simulink model "Simul_BASE_XLS"  (Simulink 9.0)
settings: Solver=FixedStepAuto  StartTime=0.0  StopTime=140  FixedStep=0.1  RelTol=1e-3  EnableMultiTasking=on
values from neighbouring files (symbols this model uses):
  attitude_0 = [0,0,0]    [ga_detumbling.m]    (also in ga_detumbling_fit.m = [0.0524,-0.0349,0.0175]; ga_pid.m; ga_pid_fit.m; ga_pid_test.m)
  attitude_rate_0 = [0,6.7e-05,0.0041]    [ga_detumbling.m]    (also in ga_detumbling_fit.m = [0.0873,-0.0873,-0.0873]; ga_pid.m; ga_pid_fit.m; ga_pid_test.m)
  dp = x(2)    [ga_detumbling.m]    (also in ga_detumbling_fit.m = d(2); ga_pid.m = x(4); ga_pid_fit.m = d(4); ga_pid_test.m = x(4))
  dr = x(1)    [ga_detumbling.m]    (also in ga_detumbling_fit.m = d(1); ga_pid.m = x(2); ga_pid_fit.m = d(2); ga_pid_test.m = x(2))
  dy = x(3)    [ga_detumbling.m]    (also in ga_detumbling_fit.m = d(3); ga_pid.m = x(6); ga_pid_fit.m = d(6); ga_pid_test.m = x(6))
  override = 2    [ga_pid_fit.m]    (also in ga_pid_test.m; init_var.m)
  pp = x(3)    [ga_pid.m]    (also in ga_pid_fit.m = d(3); ga_pid_test.m; init_var.m = 0.6885)
  pr = x(1)    [ga_pid.m]    (also in ga_pid_fit.m = d(1); ga_pid_test.m; init_var.m = 0.8646)
  py = x(5)    [ga_pid.m]    (also in ga_pid_fit.m = d(5); ga_pid_test.m; init_var.m = 0.371)
  slew = [60 0 0]    [ga_detumbling.m]    (also in ga_pid.m; ga_pid_fit.m; ga_pid_test.m)
libraries: simulink_extras x14, aerolibanim x1, sharedutil x1
CloseFcn:
  | rtwprivate ssgencode ModelCloseRequest Simul_BASE_3MW
settings Model: Creator=Kendrick  LastModifiedBy=bjt
settings SolverCC: MaxConsecutiveMinStep=5  ZeroCrossAlgorithm=Adaptive
settings DataIOCC: LimitDataPoints=on
settings OptimizationCC: ExpressionDepthLimit=2147483647
settings DebuggingCC: AlgebraicLoopMsg=none  SolverPrmCheckMsg=warning  FcnCallInpInsideContextMsg=warning  StateNameClashWarn=warning
settings HardwareCC: ProdBitPerInt=16  ProdBitPerPointer=16  ProdBitPerSizeT=16  ProdBitPerPtrDiffT=16  ProdWordSize=16  ProdHWDeviceType=Generic->16-bit Embedded Processor
settings GRTTargetCC: GeneratePreprocessorConditionals=Disable all  CombineOutputUpdateFcns=off  GRTInterface=on
settings SimscapeCC: ExplicitSolverDiagnosticOptions=error  GlobalZcOffDiagnosticOptions=error  SimscapeNormalizeSystem=off
settings SimMechanicsCC: VisOnUpdateDiagram=on  VisDuringSimulation=on  LastVizWinPosition=[824 49 610 743]  CamPosition=[0.0449883;0.218364;11.4685;]  CamTarget=[-0.000193585;-0.0218554;-0.00055518;]  CamUpVector=[-0.0100593;0.999731;-0.0208998;]  CamHeight=0.706401  VisBackgroundColor=[0.9;0.9;0.95;]  DefaultBodyColor=[1;0;0;]
settings ConfigurationSet: Description=SimMechanics 2G

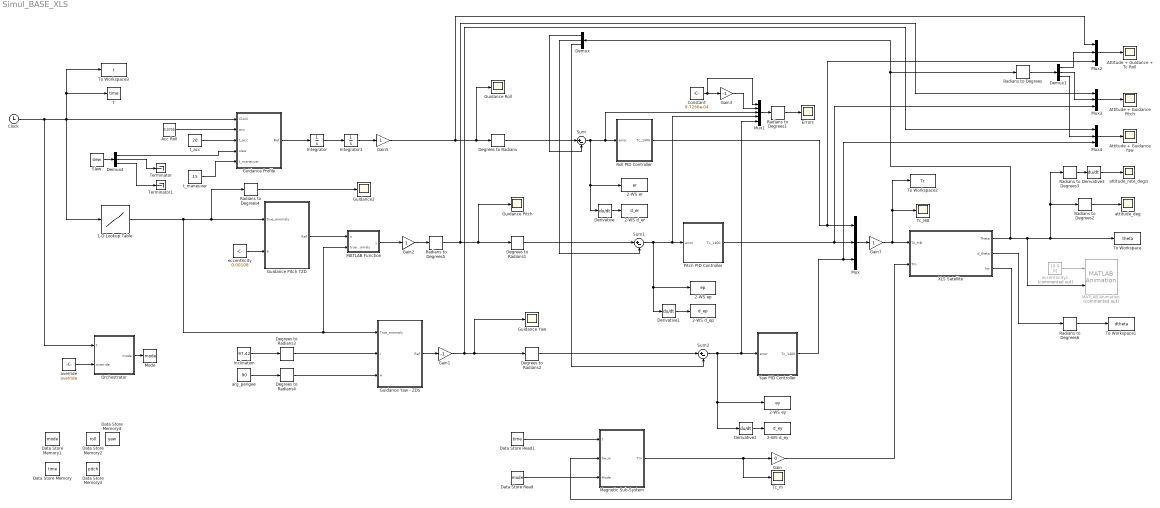
== system Simul_BASE_XLS ==
  1-D Lookup Table : Lookup_n-D  NumberOfTableDimensions=1  BreakpointsForDimension1=[0,5619.6]  Table=[0,2*pi()]  InternalRulePriority=Speed  RndMeth=Simplest  InputSameDT=on
  2-WS d_ep : ToWorkspace  VariableName=d_ep  SampleTime=-1
  2-WS d_er : ToWorkspace  VariableName=d_er  SampleTime=-1
  2-WS d_ey : ToWorkspace  VariableName=d_ey  SampleTime=-1
  2-WS ep : ToWorkspace  VariableName=ep  SampleTime=-1
  2-WS er : ToWorkspace  VariableName=er  SampleTime=-1
  2-WS ey : ToWorkspace  VariableName=ey  SampleTime=-1
  Acc Roll : Constant  Value=0.0755
  Attitude + Guidance Pitch : Scope
  Attitude + Guidance Yaw : Scope
  Attitude + Guidance + Tc Roll : Scope
  Clock : Clock
  Constant : Constant  Value=8.7266e-04
  Data Store Memory : DataStoreMemory  DataStoreName=time  ReadBeforeWriteMsg=warning  WriteAfterWriteMsg=warning  WriteAfterReadMsg=warning  ShowAdditionalParam=off
  Data Store Memory1 : DataStoreMemory  DataStoreName=mode  ReadBeforeWriteMsg=warning  WriteAfterWriteMsg=warning  WriteAfterReadMsg=warning  ShowAdditionalParam=off
  Data Store Memory2 : DataStoreMemory  DataStoreName=roll  ReadBeforeWriteMsg=warning  WriteAfterWriteMsg=warning  WriteAfterReadMsg=warning  ShowAdditionalParam=off
  Data Store Memory3 : DataStoreMemory  DataStoreName=pitch  ReadBeforeWriteMsg=warning  WriteAfterWriteMsg=warning  WriteAfterReadMsg=warning  ShowAdditionalParam=off
  Data Store Memory4 : DataStoreMemory  DataStoreName=yaw  ReadBeforeWriteMsg=warning  WriteAfterWriteMsg=warning  WriteAfterReadMsg=warning  ShowAdditionalParam=off
  Data Store Read : DataStoreRead  DataStoreName=mode
  Data Store Read1 : DataStoreRead  DataStoreName=time  DataStoreElements=time
  Degrees to Radians{,1..4} (5 alike) : simulink_extras/Transformations/Degrees to Radians
  Demux : Demux  Outputs=3
  Demux1 : Demux  Outputs=3
  Demux4 : Demux  Outputs=3
  Derivative{,1..3} (4 alike) : Derivative
  Errors : Scope
  Gain : Gain  Gain=0
  Gain1 : Gain  Gain=-1
  Gain2 : Gain
  Gain3 : Gain  Gain=-1
  Gain5 : Gain
  Gain7 : Gain
  Guidance Pitch : Scope
  Guidance Pitch TZD : MATLAB Function  TreatAsAtomicUnit=on
  Guidance Profile : MATLAB Function  TreatAsAtomicUnit=on
  Guidance Roll : Scope
  Guidance Yaw : Scope
  Guidance Yaw - ZDS : MATLAB Function  TreatAsAtomicUnit=on
  Guidance2 : Scope
  Inclination : Constant  Value=97.42
  Integrator : Integrator
  Integrator1 : Integrator
  MATLAB Animation : aerolibanim/MATLAB Animation  Tag=Matlab Animation 6 DOF  Commented=on  Vehicles=1  Geometries='XLS.mat'  BoundingBoxCoordinates=[-50,50,-50,50,-50,50]  CameraOffset=[0,0,-150]  CameraViewAngle=3  SampleTime=0.1  FigurePosition=[0,2,806,1381]
      settings: SourceProductName=Aerospace Blockset  SourceProductBaseCode=AE
  MATLAB Function : MATLAB Function  TreatAsAtomicUnit=on
  Magnetic Sub-System : Subsystem
  Mode : DataStoreWrite  DataStoreName=mode
  Mux{,2..4} (4 alike) : Mux  Inputs=3
  Mux1 : Mux  Inputs=5
  Orchestrator : MATLAB Function  TreatAsAtomicUnit=on
  Pitch PID Controller : Subsystem
  Radians to Degrees{,1..6} (7 alike) : simulink_extras/Transformations/Radians to Degrees
  Roll PID Controller : Subsystem
  Slew : Constant  Value=slew  VectorParams1D=off
  Sum : Sum  Inputs=|+-
  Sum1 : Sum  Inputs=|+-
  Sum2 : Sum  Inputs=|+-
  Tc_HB : Scope
  Tc_m : Scope
  Terminator : Terminator
  Terminator1 : Terminator
  To Workspace : ToWorkspace  VariableName=theta  SampleTime=-1
  To Workspace1 : ToWorkspace  VariableName=dtheta  SampleTime=-1
  To Workspace2 : ToWorkspace  VariableName=Tc  SampleTime=-1
  To Workspace3 : ToWorkspace  VariableName=t  SampleTime=-1
  XLS Satellite : Subsystem
  Yaw PID Controller : Subsystem
  arg_perigee : Constant  Value=90
  attitude_deg : Scope
  attitude_rate_deg/s : Scope
  eccentricity : Constant  Value=0.00108
  eccentricity1 : Constant  Commented=on  Value=[0 0 0]
  override : Constant  Value=override  VectorParams1D=off
  t : DataStoreWrite  DataStoreName=time  DataStoreElements=time
  t_acc : Constant  Value=20
  t_maneuver : Constant  Value=15
  wires:
  Sum/1 -> Mux1/3, Roll PID Controller/1(error), Derivative/1, 2-WS er/1
  Sum2/1 -> Mux1/5, Yaw PID Controller/1(error), Derivative2/1, 2-WS ey/1
  Demux/3 -> Sum2/2
  Degrees to Radians2/1 -> Sum2/1
  Demux/1 -> Sum/2
  Derivative/1 -> 2-WS d_er/1
  Derivative1/1 -> 2-WS d_ep/1
  Derivative2/1 -> 2-WS d_ey/1
  Pitch PID Controller/1(Tc_1400) -> Mux/2, Mux3/3
  XLS Satellite/2(d_theta) -> Radians to Degrees6/1
  Guidance Profile/1(Ref) -> Integrator/1
  Mux1/1 -> Radians to Degrees1/1
  Radians to Degrees1/1 -> Errors/1
  Mux2/1 -> Attitude + Guidance + Tc Roll/1
  Integrator/1 -> Integrator1/1
  Integrator1/1 -> Gain5/1
  Radians to Degrees/1 -> Demux1/1
  Demux1/1 -> Mux2/2
  Mux3/1 -> Attitude + Guidance Pitch/1
  Mux4/1 -> Attitude + Guidance Yaw/1
  Demux1/3 -> Mux4/2
  Demux1/2 -> Mux3/2
  Mux/1 -> Gain7/1
  Sum1/1 -> Derivative1/1, 2-WS ep/1, Mux1/4, Pitch PID Controller/1(error)
  Roll PID Controller/1(Tc_1400) -> Mux2/3, Mux/1
  Clock/1 -> Orchestrator/1(t), 1-D Lookup Table/1, Guidance Profile/1(Clock), To Workspace3/1, t/1
  Acc Roll/1 -> Guidance Profile/2(acc)
  eccentricity/1 -> Guidance Pitch TZD/2(e)
  Inclination/1 -> Degrees to Radians3/1
  Slew/1 -> Demux4/1
  Demux4/1 -> Guidance Profile/4(slew)
  t_acc/1 -> Guidance Profile/3(t_acc)
  arg_perigee/1 -> Degrees to Radians4/1
  Gain5/1 -> Degrees to Radians/1, Guidance Roll/1, Mux2/1
  Degrees to Radians/1 -> Sum/1
  Degrees to Radians1/1 -> Sum1/1
  Demux/2 -> Sum1/2
  XLS Satellite/3(hw) -> Magnetic Sub-System/2(hw_w)
  Gain/1 -> XLS Satellite/2(Tm)
  Gain2/1 -> Radians to Degrees5/1
  Gain7/1 -> XLS Satellite/1(Tc_HB), To Workspace2/1, Tc_HB/1
  Derivative3/1 -> attitude_rate_deg/s/1
  Radians to Degrees2/1 -> attitude_deg/1
  Radians to Degrees3/1 -> Derivative3/1
  Magnetic Sub-System/1(Tm) -> Tc_m/1, Gain/1
  Yaw PID Controller/1(Tc_1400) -> Mux4/3, Mux/3
  Data Store Read1/1 -> Magnetic Sub-System/1(t)
  Orchestrator/1(mode) -> Mode/1
  override/1 -> Orchestrator/2(override)
  Data Store Read/1 -> Magnetic Sub-System/3(Mode)
  XLS Satellite/1(Theta) -> MATLAB Animation/2, To Workspace/1, Radians to Degrees2/1, Radians to Degrees3/1, Demux/1, Radians to Degrees/1
  Gain1/1 -> Guidance Yaw/1, Degrees to Radians2/1, Mux4/1
  1-D Lookup Table/1 -> Radians to Degrees4/1, Guidance Pitch TZD/1(true_anomaly), Guidance Yaw - ZDS/1(True_anomaly), MATLAB Function/2(true_anomaly)
  Radians to Degrees4/1 -> Guidance2/1
  Demux4/2 -> Terminator/1
  Demux4/3 -> Terminator1/1
  Degrees to Radians3/1 -> Guidance Yaw - ZDS/2(i)
  Guidance Yaw - ZDS/1(Ref) -> Gain1/1
  Degrees to Radians4/1 -> Guidance Yaw - ZDS/3(w)
  Guidance Pitch TZD/1(Ref) -> MATLAB Function/1(u)
  MATLAB Function/1(y) -> Gain2/1
  Radians to Degrees5/1 -> Guidance Pitch/1, Degrees to Radians1/1, Mux3/1
  t_maneuver/1 -> Guidance Profile/5(t_maneuver)
  eccentricity1/1 -> MATLAB Animation/1
  Radians to Degrees6/1 -> To Workspace1/1
  Constant/1 -> Mux1/1, Gain3/1
  Gain3/1 -> Mux1/2

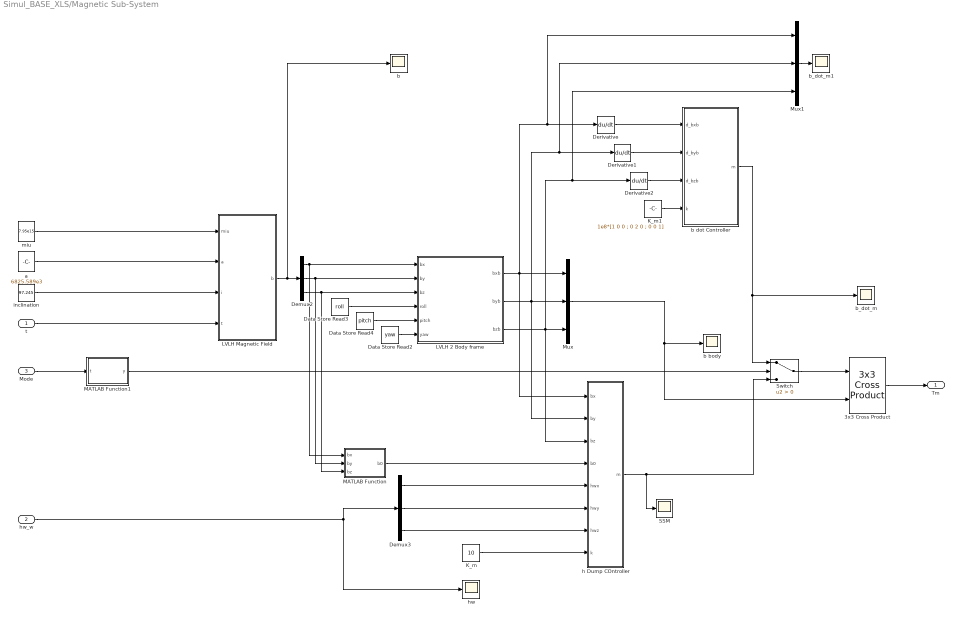
== system Simul_BASE_XLS/Magnetic Sub-System ==
  t : Inport
  hw_w : Inport  Port=2
  Mode : Inport  Port=3
  3x3 Cross Product : sharedutil/3x3 Cross Product
      settings: SourceProductBaseCode=AE
  Data Store Read2 : DataStoreRead  DataStoreName=yaw
  Data Store Read3 : DataStoreRead  DataStoreName=roll
  Data Store Read4 : DataStoreRead  DataStoreName=pitch
  Demux2 : Demux  Outputs=3
  Demux3 : Demux  Outputs=3
  Derivative : Derivative
  Derivative1 : Derivative
  Derivative2 : Derivative
  K_m : Constant  Value=10
  K_m1 : Constant  Value=1e8*[1 0 0 ; 0 2 0 ; 0 0 1]
  LVLH 2 Body frame : MATLAB Function  TreatAsAtomicUnit=on
  LVLH Magnetic Field : MATLAB Function  TreatAsAtomicUnit=on
  MATLAB Function : MATLAB Function  TreatAsAtomicUnit=on
  MATLAB Function1 : MATLAB Function  TreatAsAtomicUnit=on
  Mux : Mux  Inputs=3
  Mux1 : Mux  Inputs=3
  SSM : Scope
  Switch : Switch  Criteria=u2 > Threshold
  a : Constant  Value=6825.589e3
  b : Scope
  b body : Scope
  b dot Controller : MATLAB Function  TreatAsAtomicUnit=on
  b_dot_m : Scope
  b_dot_m1 : Scope
  h Dump COntroller : MATLAB Function  TreatAsAtomicUnit=on
  hw : Scope
  inclination : Constant  Value=97.245
  miu : Constant  Value=7.95e15
  Tm : Outport
  wires:
  Demux3/3 -> h Dump COntroller/7(hwz)
  hw_w/1 -> hw/1, Demux3/1
  Demux3/2 -> h Dump COntroller/6(hwy)
  inclination/1 -> LVLH Magnetic Field/3(i)
  t/1 -> LVLH Magnetic Field/4(t)
  Demux2/1 -> MATLAB Function/1(bx), LVLH 2 Body frame/1(bx)
  Demux2/2 -> MATLAB Function/2(by), LVLH 2 Body frame/2(by)
  Demux2/3 -> MATLAB Function/3(bz), LVLH 2 Body frame/3(bz)
  LVLH Magnetic Field/1(b) -> Demux2/1, b/1
  miu/1 -> LVLH Magnetic Field/1(miu)
  K_m/1 -> h Dump COntroller/8(k)
  Demux3/1 -> h Dump COntroller/5(hwx)
  a/1 -> LVLH Magnetic Field/2(a)
  MATLAB Function/1(b0) -> h Dump COntroller/4(b0)
  K_m1/1 -> b dot Controller/4(k)
  Mode/1 -> MATLAB Function1/1(t)
  Derivative/1 -> b dot Controller/1(d_bxb)
  Derivative1/1 -> b dot Controller/2(d_byb)
  Derivative2/1 -> b dot Controller/3(d_bzb)
  Switch/1 -> 3x3 Cross Product/1
  Mux/1 -> b body/1, 3x3 Cross Product/2
  h Dump COntroller/1(m) -> SSM/1, Switch/3
  b dot Controller/1(m) -> Switch/1, b_dot_m/1
  3x3 Cross Product/1 -> Tm/1
  MATLAB Function1/1(y) -> Switch/2
  Data Store Read3/1 -> LVLH 2 Body frame/4(roll)
  Data Store Read4/1 -> LVLH 2 Body frame/5(pitch)
  Data Store Read2/1 -> LVLH 2 Body frame/6(yaw)
  LVLH 2 Body frame/1(bxb) -> h Dump COntroller/1(bx), Mux1/1, Derivative/1, Mux/1
  LVLH 2 Body frame/2(byb) -> h Dump COntroller/2(by), Mux1/2, Derivative1/1, Mux/2
  LVLH 2 Body frame/3(bzb) -> h Dump COntroller/3(bz), Mux1/3, Derivative2/1, Mux/3
  Mux1/1 -> b_dot_m1/1

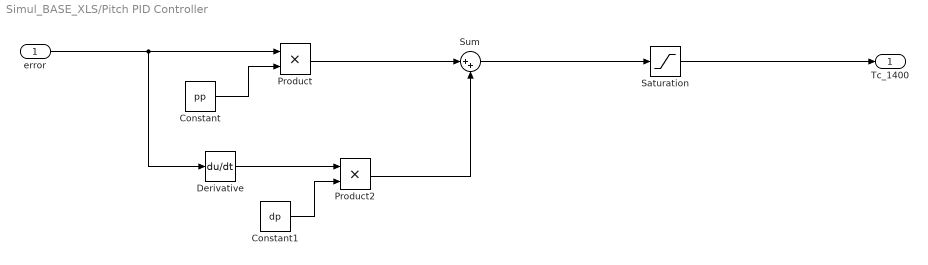
== system Simul_BASE_XLS/Pitch PID Controller ==
  error : Inport
  Constant : Constant  Value=pp
  Constant1 : Constant  Value=dp
  Derivative : Derivative
  Product : Product
  Product2 : Product
  Saturation : Saturate  UpperLimit=1.2929  LowerLimit=-1.2929
  Sum : Sum  Inputs=|++
  Tc_1400 : Outport
  wires:
  Sum/1 -> Saturation/1
  Product2/1 -> Sum/2
  Product/1 -> Sum/1
  Constant/1 -> Product/2
  Constant1/1 -> Product2/2
  Derivative/1 -> Product2/1
  error/1 -> Derivative/1, Product/1
  Saturation/1 -> Tc_1400/1

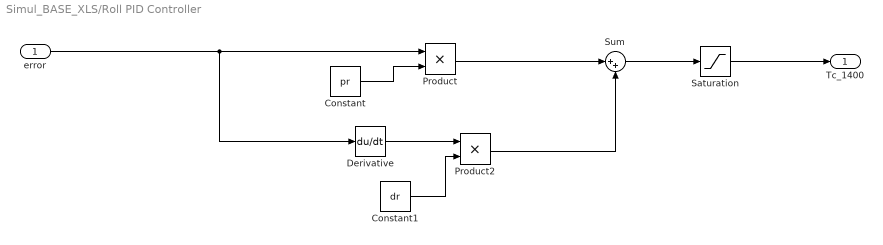
== system Simul_BASE_XLS/Roll PID Controller ==
  error : Inport
  Constant : Constant  Value=pr
  Constant1 : Constant  Value=dr
  Derivative : Derivative
  Product : Product
  Product2 : Product
  Saturation : Saturate  UpperLimit=0.6929  LowerLimit=-0.6929
  Sum : Sum  Inputs=|++
  Tc_1400 : Outport
  wires:
  Sum/1 -> Saturation/1
  Product2/1 -> Sum/2
  Product/1 -> Sum/1
  Constant/1 -> Product/2
  Constant1/1 -> Product2/2
  Derivative/1 -> Product2/1
  Saturation/1 -> Tc_1400/1
  error/1 -> Derivative/1, Product/1

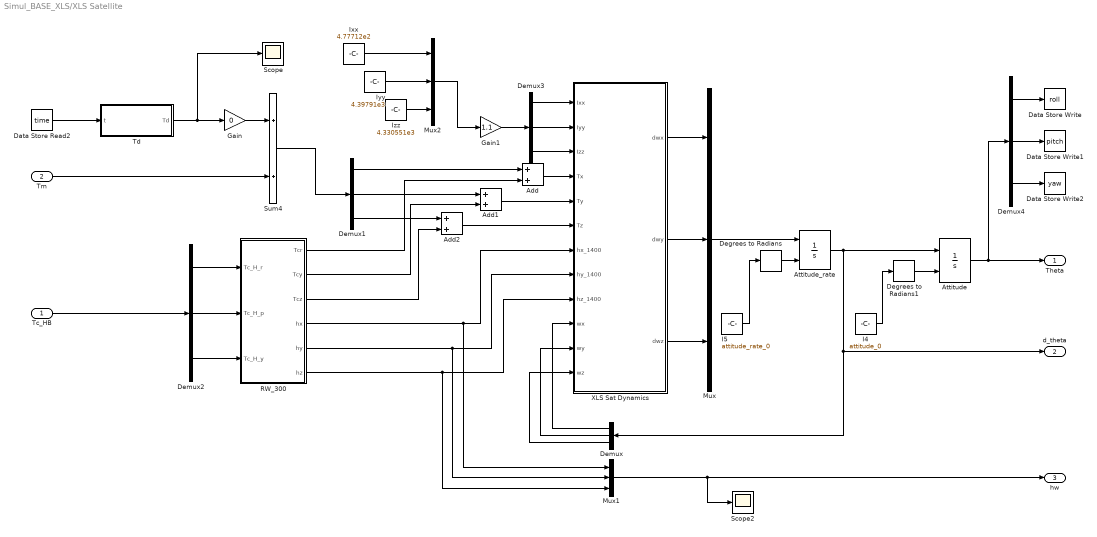
== system Simul_BASE_XLS/XLS Satellite ==
  Tc_HB : Inport
  Tm : Inport  Port=2
  Add : Sum
  Add1 : Sum
  Add2 : Sum
  Attitude : Integrator  InitialConditionSource=external
  Attitude_rate : Integrator  InitialConditionSource=external
  Data Store Read2 : DataStoreRead  DataStoreName=time
  Data Store Write : DataStoreWrite  DataStoreName=roll
  Data Store Write1 : DataStoreWrite  DataStoreName=pitch
  Data Store Write2 : DataStoreWrite  DataStoreName=yaw
  Degrees to Radians : simulink_extras/Transformations/Degrees to Radians
  Degrees to Radians1 : simulink_extras/Transformations/Degrees to Radians
  Demux{,1..4} (5 alike) : Demux  Outputs=3
  Gain : Gain  Gain=0
  Gain1 : Gain  Gain=1.1
  I4 : Constant  Value=attitude_0
  I5 : Constant  Value=attitude_rate_0
  Ixx : Constant  Value=4.77712e2
  Iyy : Constant  Value=4.39791e3
  Izz : Constant  Value=4.330551e3
  Mux : Mux  Inputs=3
  Mux1 : Mux  Inputs=3
  Mux2 : Mux  Inputs=3
  RW_300 : Subsystem
  Scope : Scope
  Scope2 : Scope
  Sum4 : Sum
  Td : Subsystem
  XLS Sat Dynamics : MATLAB Function  TreatAsAtomicUnit=on
  Theta : Outport
  d_theta : Outport  Port=2
  hw : Outport  Port=3
  wires:
  Data Store Read2/1 -> Td/1(t)
  Attitude/1 -> Demux4/1, Theta/1
  Attitude_rate/1 -> Attitude/1, Demux/1, d_theta/1
  Demux/1 -> XLS Sat Dynamics/10(wx)
  Demux/2 -> XLS Sat Dynamics/11(wy)
  Demux/3 -> XLS Sat Dynamics/12(wz)
  XLS Sat Dynamics/1(dwx) -> Mux/1
  XLS Sat Dynamics/2(dwy) -> Mux/2
  XLS Sat Dynamics/3(dwz) -> Mux/3
  Mux/1 -> Attitude_rate/1
  Td/1(Td) -> Scope/1, Gain/1
  Tm/1 -> Sum4/2
  Mux1/1 -> Scope2/1, hw/1
  Tc_HB/1 -> Demux2/1
  I4/1 -> Degrees to Radians1/1
  I5/1 -> Degrees to Radians/1
  Degrees to Radians/1 -> Attitude_rate/2
  Degrees to Radians1/1 -> Attitude/2
  Sum4/1 -> Demux1/1
  Gain/1 -> Sum4/1
  Demux4/1 -> Data Store Write/1
  Demux4/2 -> Data Store Write1/1
  Demux4/3 -> Data Store Write2/1
  Demux2/1 -> RW_300/1(Tc_H_r)
  Demux2/2 -> RW_300/2(Tc_H_p)
  Demux2/3 -> RW_300/3(Tc_H_y)
  RW_300/1(Tcr) -> Add/2
  Add/1 -> XLS Sat Dynamics/4(Tx)
  Demux1/1 -> Add/1
  RW_300/2(Tcy) -> Add1/2
  Demux1/2 -> Add1/1
  Add1/1 -> XLS Sat Dynamics/5(Ty)
  Add2/1 -> XLS Sat Dynamics/6(Tz)
  RW_300/3(Tcz) -> Add2/2
  Demux1/3 -> Add2/1
  RW_300/4(hx) -> Mux1/1, XLS Sat Dynamics/7(hx_1400)
  RW_300/5(hy) -> Mux1/2, XLS Sat Dynamics/8(hy_1400)
  RW_300/6(hz) -> Mux1/3, XLS Sat Dynamics/9(hz_1400)
  Demux3/3 -> XLS Sat Dynamics/3(Izz)
  Demux3/2 -> XLS Sat Dynamics/2(Iyy)
  Demux3/1 -> XLS Sat Dynamics/1(Ixx)
  Gain1/1 -> Demux3/1
  Mux2/1 -> Gain1/1
  Ixx/1 -> Mux2/1
  Izz/1 -> Mux2/3
  Iyy/1 -> Mux2/2

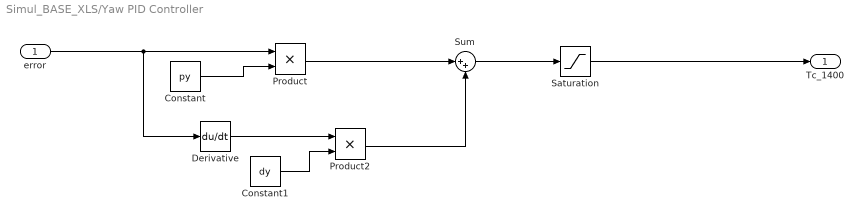
== system Simul_BASE_XLS/Yaw PID Controller ==
  error : Inport
  Constant : Constant  Value=py
  Constant1 : Constant  Value=dy
  Derivative : Derivative
  Product : Product
  Product2 : Product
  Saturation : Saturate  UpperLimit=0.6929  LowerLimit=-0.6929
  Sum : Sum  Inputs=|++
  Tc_1400 : Outport
  wires:
  Sum/1 -> Saturation/1
  Product2/1 -> Sum/2
  Product/1 -> Sum/1
  Constant/1 -> Product/2
  Constant1/1 -> Product2/2
  Derivative/1 -> Product2/1
  error/1 -> Product/1, Derivative/1
  Saturation/1 -> Tc_1400/1

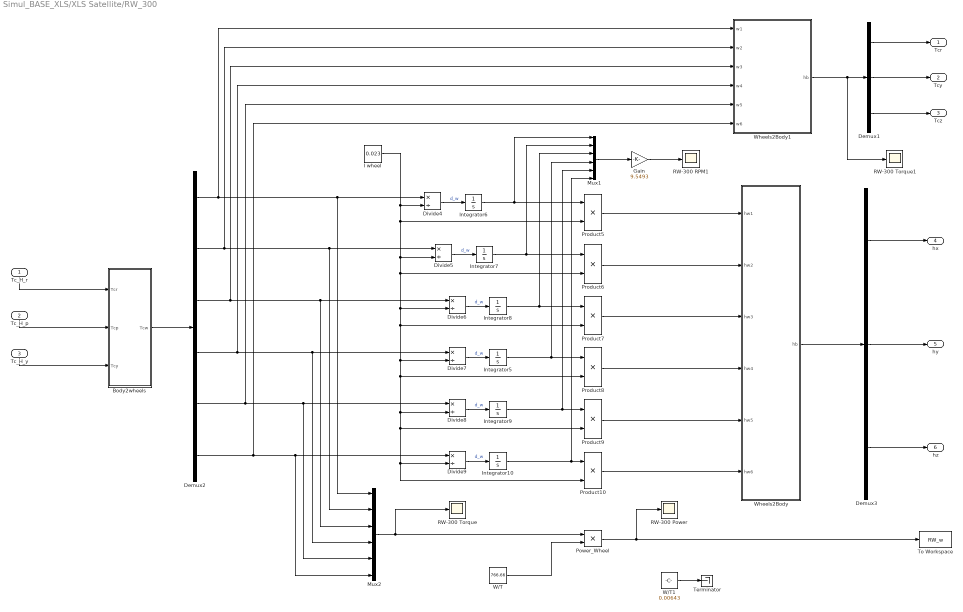
== system Simul_BASE_XLS/XLS Satellite/RW_300 ==
  Tc_H_r : Inport
  Tc_H_p : Inport  Port=2
  Tc_H_y : Inport  Port=3
  Body2wheels : MATLAB Function  TreatAsAtomicUnit=on
  Demux1 : Demux  Outputs=3
  Demux2 : Demux  Outputs=6
  Demux3 : Demux  Outputs=3
  Divide{4..9} (6 alike) : Product  Inputs=*/
  Gain : Gain  Gain=9.5493
  I wheel : Constant  Value=0.023
  Integrator{5..10} (6 alike) : Integrator
  Mux1 : Mux  Inputs=6
  Mux2 : Mux  Inputs=6
  Power_Wheel : Product  Inputs=**
  Product{5..10} (6 alike) : Product
  RW-300 Power : Scope
  RW-300 RPM1 : Scope
  RW-300 Torque : Scope
  RW-300 Torque1 : Scope
  Terminator : Terminator
  To Workspace : ToWorkspace  VariableName=RW_w  SampleTime=-1
  W/T : Constant  Value=766.66
  W/T1 : Constant  Value=0.00643
  Wheels2Body : MATLAB Function  TreatAsAtomicUnit=on
  Wheels2Body1 : MATLAB Function  TreatAsAtomicUnit=on
  Tcr : Outport
  Tcy : Outport  Port=2
  Tcz : Outport  Port=3
  hx : Outport  Port=4
  hy : Outport  Port=5
  hz : Outport  Port=6
  wires:
  Divide5/1 -> Integrator7/1  "d_w"
  Mux1/1 -> Gain/1
  Product9/1 -> Wheels2Body/5(hw5)
  W/T1/1 -> Terminator/1
  Demux2/3 -> Wheels2Body1/3(w3), Divide6/1, Mux2/3
  Demux2/1 -> Wheels2Body1/1(w1), Divide4/1, Mux2/1
  Integrator5/1 -> Mux1/4, Product8/1
  Power_Wheel/1 -> RW-300 Power/1, To Workspace/1
  W/T/1 -> Power_Wheel/2
  Integrator10/1 -> Mux1/6, Product10/1
  Product5/1 -> Wheels2Body/1(hw1)
  I wheel/1 -> Product5/2, Product6/2, Product10/2, Divide9/2, Product9/2, Divide8/2, Product8/2, Divide7/2, Product7/2, Divide6/2, Divide5/2, Divide4/2
  Integrator7/1 -> Product6/1, Mux1/2
  Gain/1 -> RW-300 RPM1/1
  Integrator6/1 -> Product5/1, Mux1/1
  Tc_H_y/1 -> Body2wheels/3(Tcy)
  Wheels2Body/1(hb) -> Demux3/1
  Product7/1 -> Wheels2Body/3(hw3)
  Demux2/6 -> Wheels2Body1/6(w6), Mux2/6, Divide9/1
  Demux2/4 -> Wheels2Body1/4(w4), Divide7/1, Mux2/4
  Tc_H_r/1 -> Body2wheels/1(Tcr)
  Product6/1 -> Wheels2Body/2(hw2)
  Integrator9/1 -> Mux1/5, Product9/1
  Body2wheels/1(Tcw) -> Demux2/1
  Divide9/1 -> Integrator10/1  "d_w"
  Divide8/1 -> Integrator9/1  "d_w"
  Tc_H_p/1 -> Body2wheels/2(Tcp)
  Mux2/1 -> RW-300 Torque/1, Power_Wheel/1
  Divide4/1 -> Integrator6/1  "d_w"
  Product8/1 -> Wheels2Body/4(hw4)
  Divide6/1 -> Integrator8/1  "d_w"
  Product10/1 -> Wheels2Body/6(hw6)
  Demux2/5 -> Wheels2Body1/5(w5), Divide8/1, Mux2/5
  Integrator8/1 -> Mux1/3, Product7/1
  Divide7/1 -> Integrator5/1  "d_w"
  Demux2/2 -> Wheels2Body1/2(w2), Divide5/1, Mux2/2
  Wheels2Body1/1(hb) -> Demux1/1, RW-300 Torque1/1
  Demux1/1 -> Tcr/1
  Demux1/2 -> Tcy/1
  Demux1/3 -> Tcz/1
  Demux3/1 -> hx/1
  Demux3/2 -> hy/1
  Demux3/3 -> hz/1

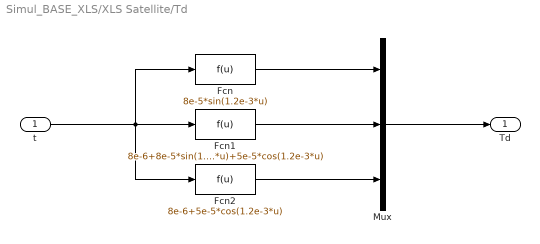
== system Simul_BASE_XLS/XLS Satellite/Td ==
  t : Inport
  Fcn : Fcn  Expr=8e-5*sin(1.2e-3*u)
  Fcn1 : Fcn  Expr=8e-6+8e-5*sin(1.2e-3*u)+5e-5*cos(1.2e-3*u)
  Fcn2 : Fcn  Expr=8e-6+5e-5*cos(1.2e-3*u)
  Mux : Mux  Inputs=3
  Td : Outport
  wires:
  t/1 -> Fcn1/1, Fcn/1, Fcn2/1
  Fcn1/1 -> Mux/2
  Fcn/1 -> Mux/1
  Fcn2/1 -> Mux/3
  Mux/1 -> Td/1

== matlab function XLS Satellite/XLS Sat Dynamics ==
  data: Ixx input double; Iyy input double; Izz input double; Tx input double; Ty input double; Tz input double; hx_1400 input double; hy_1400 input double; hz_1400 input double; wx input double; wy input double; wz input double; dwx output double; dwy output double; dwz output double
function [dwx,dwy,dwz] = Satellite(Ixx,Iyy,Izz,Tx,Ty,Tz,hx_1400,hy_1400,hz_1400,wx,wy,wz)

dwx = (Tx-(Iyy-Izz)*wz*wy+(hz_1400)*wy-(hy_1400)*wz)/Ixx;
dwy = (Ty-(Izz-Ixx)*wx*wz+(hx_1400)*wz-(hz_1400)*wx)/Iyy;
dwz = (Tz-(Ixx-Iyy)*wy*wx+(hy_1400)*wx-(hx_1400)*wy)/Izz;

== matlab function Guidance Profile ==
  data: Clock input double; Ref output double; acc input double; t_acc input double; slew input double; t_maneuver input double
function Ref = Slew_Guidance(Clock,acc,t_acc,slew,t_maneuver)
u=0;
if Clock>=t_maneuver
    t_c=(slew/acc-t_acc^2)/t_acc;

    if Clock<t_acc+t_maneuver
        u=acc;
    end

    if Clock>=t_acc+t_c+t_maneuver&&Clock<2*t_acc+t_c+t_maneuver
        u=-acc;
    end
    if slew==0
        Ref = 0;
    else
        Ref = u;
    end
else
Ref=0;
end

== matlab function Guidance Pitch TZD ==
  data: true_anomaly input double; Ref output double; e input double
function Ref = TZDS(true_anomaly,e)
Ref=(1+e*cos(true_anomaly))/(sqrt(1+e^2+2*e*cos(true_anomaly)));

== matlab function Guidance Yaw - ZDS ==
  data: True_anomaly input double; Ref output double; i input double; w input double
function Ref= ZDS(True_anomaly,i,w)
Ref=rad2deg(atan((sin(i)*cos(w+True_anomaly))/(15.375-cos(i))));

== matlab function MATLAB Function ==
  data: u input double; y output double; true_anomaly input double
function y = fcn(u,true_anomaly)
if true_anomaly>=0&&true_anomaly<pi()
    y = acos(u);
else
    y=-acos(u);
end

== matlab function XLS Satellite/RW_300/Wheels2Body1 ==
  data: w1 input double; hb output double; w2 input double; w3 input double; w4 input double; w5 input double; w6 input double
function hb = wheels2body(w1,w2,w3,w4,w5,w6)
hb=   [ -0.5774         0   -0.5774    0.5774         0    0.5774
        -0.5774         1    0.5774    0.5774        -1   -0.5774
        -0.5774         0   -0.5774   -0.5774         0   -0.5774]*[w1;w2;w3;w4;w5;w6];

== matlab function XLS Satellite/RW_300/Body2wheels ==
  data: Tcr input double; Tcw output double; Tcp input double; Tcy input double
function Tcw = body2wheels(Tcr,Tcp,Tcy)

    Tcw= [-0.4330   -0.1732   -0.4330
           0         0.3000    0
          -0.4330    0.1732   -0.4330
           0.4330    0.1732   -0.4330
           0        -0.3000    0
           0.4330   -0.1732   -0.4330]*[Tcr;Tcp;Tcy];

== matlab function XLS Satellite/RW_300/Wheels2Body ==
  data: hw1 input double; hb output double; hw2 input double; hw3 input double; hw4 input double; hw5 input double; hw6 input double
function hb = wheels2body(hw1,hw2,hw3,hw4,hw5,hw6)
hb=   [ -0.5774         0   -0.5774    0.5774         0    0.5774
        -0.5774         1    0.5774    0.5774        -1   -0.5774
        -0.5774         0   -0.5774   -0.5774         0   -0.5774]*[hw1;hw2;hw3;hw4;hw5;hw6];

== matlab function Magnetic Sub-System/LVLH 2 Body frame ==
  data: bx input double; bxb output double; by input double; bz input double; roll input double; pitch input double; yaw input double; byb output double; bzb output double
function [bxb,byb,bzb] = fcn(bx,by,bz,roll,pitch,yaw)
bb=[cos(pitch)          ,-cos(yaw)*sin(pitch)                               ,sin(pitch)*sin(yaw);
    cos(roll)*sin(pitch), cos(roll)*cos(pitch)*cos(yaw)-sin(roll)*sin(yaw)  ,-cos(yaw)*sin(roll)-cos(roll)*cos(pitch)*sin(yaw);
    sin(roll)*sin(pitch), cos(roll)*sin(yaw)+cos(pitch)*cos(yaw)*sin(roll)   , cos(roll)*cos(yaw)-cos(pitch)*sin(roll)*sin(yaw)]*[bx;by;bz];
bxb=bb(1);
byb=bb(2);
bzb=bb(3);

== matlab function Magnetic Sub-System/h Dump COntroller ==
  data: bx input double; by input double; bz input double; b0 input double; hwx input double; hwy input double; hwz input double; k input double; m output double
function m  = fcn(bx,by,bz,b0,hwx, hwy, hwz,k)
m=-k/b0^2*cross([bx ; by ; bz] ,[hwx;hwy;hwz]);
for i=1:3
    if m(i)>110||m(i)<-100
        m(i)=110;
    end
end
%cross(m,[bxb ; byb ; bzb]);

== matlab function Magnetic Sub-System/LVLH Magnetic Field ==
  data: miu input double; a input double; i input double; b output double; t input double
function b = magnetic_field(miu,a,i,t)

b = miu/a^3*[sin(deg2rad(i))*cos(1.2e-3*t);
    -cos(deg2rad(i));
    2*sin(deg2rad(i))*sin(1.2e-3*t)];

== matlab function Magnetic Sub-System/b dot Controller ==
  data: d_bxb input double; d_byb input double; d_bzb input double; k input double; m output double
function m = fcn(d_bxb, d_byb, d_bzb, k)
m=-k*[d_bxb ;d_byb ;d_bzb];
for i=1:3
    if m(i)>110
        m(i)=110;
    end
    if m(i)<-110
        m(i)=-110;
    end
end
%cross(m,[bxb ; byb ; bzb]);

== matlab function Magnetic Sub-System/MATLAB Function1 ==
  data: t input double; y output double
function y = fcn(t)
y=1;
if t>=10000
    y=-1;
end

== matlab function Magnetic Sub-System/MATLAB Function ==
  data: bx input double; b0 output double; by input double; bz input double
function b0 = norm(bx,by,bz)

b0 = sqrt(bx^2+by^2+bz^2);

== matlab function Orchestrator ==
  data: t input double; mode output double; override input double
function mode = mode_selector(t,override)
mode=0;
if override~=0
    mode=override;
else    
    if t==0
        mode=0;
    end
    if t>15
        mode=1;
    end
end
